simulink model "Reglung"  (R2023a)
settings: Solver=VariableStepAuto  StartTime=0.0  StopTime=inf  RelTol=1e-3
undefined symbols (not defined in the file): LF
libraries: instrumentseriallib x2
settings Model: Creator=ASUS-VivoBook  LastModifiedBy=karim

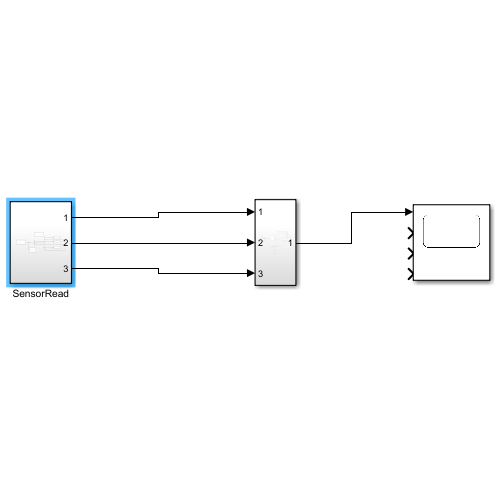
[thumbnail: Simulink's stored preview of the top-level diagram]
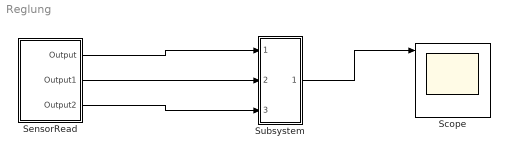
== system Reglung ==
  Scope : Scope  NumInputPorts=4
  SensorRead : Subsystem
  Subsystem : Subsystem
  wires:
  SensorRead/1(Output) -> Subsystem/1(Input)
  SensorRead/2(Output1) -> Subsystem/2(Input1)
  SensorRead/3(Output2) -> Subsystem/3(Input2)
  Subsystem/1(Out1) -> Scope/1

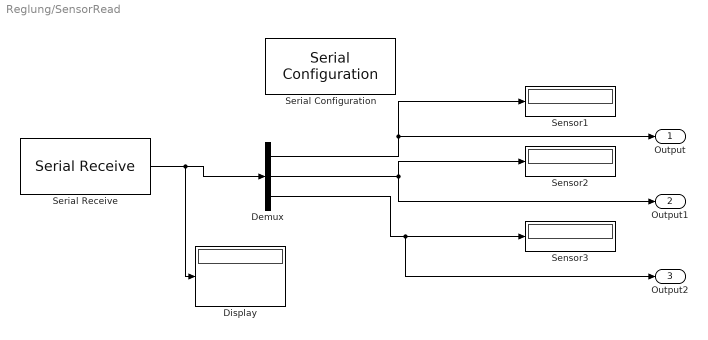
== system Reglung/SensorRead ==
  Demux : Demux  Outputs=3
  Display : Display
      settings: Decimation=3
  Sensor1 : Display
  Sensor2 : Display
  Sensor3 : Display
  Serial Configuration : instrumentseriallib/Serial Configuration  Priority=-200000  PortSel=COM7  Port=COM7  ComPort=COM7  BaudRate=115200  DataBits=8  Parity=none  StopBits=1  ByteOrder=little-endian  FlowControl=none  Timeout=10  SimulateUsing=Interpreted execution  BlockInModel=on  aMode=1
  Serial Receive : instrumentseriallib/Serial Receive  Priority=1  PortSel=COM7  Port=COM7  ComPort=COM7  DataType=single  SaveDataType=uint8  ToggleHeader=on  Header=[65]  ToggleTerminator=on  Terminator=LF ('\n')  CustomTerminator=[]  InputFormat=Column major  ToggleDataSize=on  DataSize=[1 3]  EnableBlockingMode=on  ActionDataUnavailable=Output last received value  ActionWhenDataUnavailable=Output last received value  CustomValue=0  SampleTime=0.05  SimulateUsing=Interpreted execution  BlockInModel=on  aMode=1
  Output : Outport
  Output1 : Outport  Port=2
  Output2 : Outport  Port=3
  wires:
  Demux/2 -> Sensor2/1, Output1/1
  Demux/3 -> Output2/1, Sensor3/1
  Demux/1 -> Sensor1/1, Output/1
  Serial Receive/1 -> Display/1, Demux/1

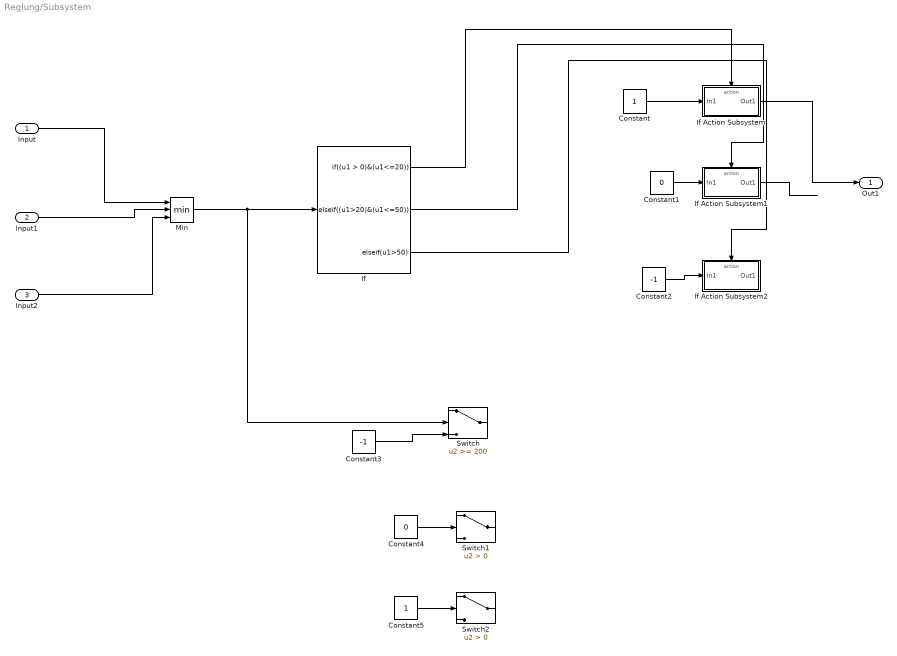
== system Reglung/Subsystem ==
  Input : Inport
  Input1 : Inport  Port=2
  Input2 : Inport  Port=3
  Constant : Constant
  Constant1 : Constant  Value=0
  Constant2 : Constant  Value=-1
  Constant3 : Constant  Value=-1
  Constant4 : Constant  Value=0
  Constant5 : Constant
  If : If  IfExpression=(u1 > 0)&(u1<=20)  ElseIfExpressions=(u1>20)&(u1<=50),u1>50  ShowElse=off
  If Action Subsystem : Subsystem  TreatAsAtomicUnit=on
  If Action Subsystem1 : Subsystem  TreatAsAtomicUnit=on
  If Action Subsystem2 : Subsystem  TreatAsAtomicUnit=on
  Min : MinMax  Inputs=3
  Switch : Switch  Threshold=200  SaturateOnIntegerOverflow=off  InputSameDT=off
  Switch1 : Switch  Criteria=u2 > Threshold  SaturateOnIntegerOverflow=off  InputSameDT=off
  Switch2 : Switch  Criteria=u2 > Threshold  SaturateOnIntegerOverflow=off  InputSameDT=off
  Out1 : Outport
  wires:
  If/1 -> If Action Subsystem/Action
  If/3 -> If Action Subsystem2/Action
  Input/1 -> Min/1
  If/2 -> If Action Subsystem1/Action
  Input1/1 -> Min/2
  Constant/1 -> If Action Subsystem/1(In1)
  Input2/1 -> Min/3
  Constant2/1 -> If Action Subsystem2/1(In1)
  Constant1/1 -> If Action Subsystem1/1(In1)
  If Action Subsystem1/1(Out1) -> ?
  If Action Subsystem/1(Out1) -> Out1/1
  Min/1 -> Switch/2, If/1
  Constant4/1 -> Switch1/2
  Constant5/1 -> Switch2/2
  Constant3/1 -> Switch/3

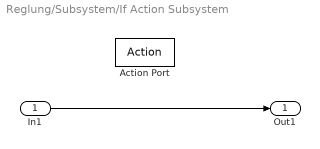
== system Reglung/Subsystem/If Action Subsystem ==
  In1 : Inport
  Action Port : ActionPort  ActionPortLabel=if((u1 > 0)&(u1<=20))
  Out1 : Outport
  wires:
  In1/1 -> Out1/1

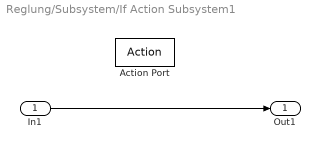
== system Reglung/Subsystem/If Action Subsystem1 ==
  In1 : Inport
  Action Port : ActionPort  ActionPortLabel=elseif((u1>20)&(u1<=50))
  Out1 : Outport
  wires:
  In1/1 -> Out1/1

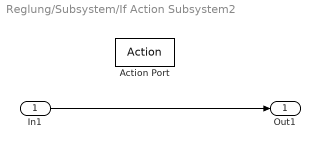
== system Reglung/Subsystem/If Action Subsystem2 ==
  In1 : Inport
  Action Port : ActionPort  ActionPortLabel=elseif(u1>50)
  Out1 : Outport
  wires:
  In1/1 -> Out1/1
